simulink model "Simscape_Model_2018b"  (R2018b)
settings: Solver=ode14x  StartTime=0.0  StopTime=timeDuration  FixedStep=TimeStamp  RelTol=1e-3
values from neighbouring files (symbols this model uses):
  N = length(Points(1,:))    [Quaternion_Simulink_Model.m]
undefined symbols (not defined in the file or in its folder): sigbuilder_block, X, Y, Z
libraries: nesl_utility x31, sm_lib x27
(part 2 of 2)

== matlab function Simscape_Model_2018b/Transformation Matrix & Position/MATLAB Function ==
  data: th1 input; transform output; th2 input; th3 input; th4 input; th5 input; th6 input
function transform = getTransformationMatrix(th1,th2,th3,th4,th5,th6)   

A1 = 0.02;      D1 = 0.345;       AL1 = pi/2;   
A2 = 0.260;     D2 = 0;           AL2 = 0;     
A3 = 0.02;      D3 = 0;           AL3 = pi/2;  
A4 = 0;         D4 = 0.260;       AL4 =-pi/2;  
A5 = 0;         D5 = 0;           AL5 = pi/2;  
A6 = 0;         D6 = 0.075;       AL6 = 0;


Eular_Rot_Mat_1 = [cos(th1)     -sin(th1)*cos(AL1)     sin(th1)*sin(AL1)     A1*cos(th1);
                   sin(th1)      cos(th1)*cos(AL1)    -cos(th1)*sin(AL1)     A1*sin(th1);
                   0             sin(AL1)              cos(AL1)              D1;
                   0             0                     0                     1];

Eular_Rot_Mat_2 = [cos(th2)     -sin(th2)*cos(AL2)     sin(th2)*sin(AL2)     A2*cos(th2);
                   sin(th2)      cos(th2)*cos(AL2)    -cos(th2)*sin(AL2)     A2*sin(th2);
                   0             sin(AL2)              cos(AL2)              D2;
                   0             0                     0                     1];
Eular_Rot_Mat_3 = [cos(th3)     -sin(th3)*cos(AL3)     sin(th3)*sin(AL3)     A3*cos(th3);
                   sin(th3)      cos(th3)*cos(AL3)    -cos(th3)*sin(AL3)     A3*sin(th3);
                   0             sin(AL3)              cos(AL3)              D3;
                   0             0                     0                     1];
Eular_Rot_Mat_4 = [cos(th4)     -sin(th4)*cos(AL4)     sin(th4)*sin(AL4)     A4*cos(th4);
                   sin(th4)      cos(th4)*cos(AL4)    -cos(th4)*sin(AL4)     A4*sin(th4);
                   0             sin(AL4)              cos(AL4)              D4;
                   0             0                     0                     1];
Eular_Rot_Mat_5 = [cos(th5)     -sin(th5)*cos(AL5)     sin(th5)*sin(AL5)     A5*cos(th5);
                   sin(th5)      cos(th5)*cos(AL5)    -cos(th5)*sin(AL5)     A5*sin(th5);
                   0             sin(AL5)              cos(AL5)              D5;
                   0             0                     0                     1];
Eular_Rot_Mat_6 = [cos(th6)     -sin(th6)*cos(AL6)     sin(th6)*sin(AL6)     A6*cos(th6);
                   sin(th6)      cos(th6)*cos(AL6)    -cos(th6)*sin(AL6)     A6*sin(th6);
                   0             sin(AL6)              cos(AL6)              D6;
                   0             0                     0                     1];
            
transform = Eular_Rot_Mat_1 * Eular_Rot_Mat_2 * Eular_Rot_Mat_3 * Eular_Rot_Mat_4 * Eular_Rot_Mat_5 * Eular_Rot_Mat_6;

end
